simulink model "System_HybridMotorcycle_v1_Wit"  (R2014a)
settings: Solver=ode15s  StartTime=0.0  StopTime=100  RelTol=1e-3
InitFcn:
  | HybridOn=30;
  | SpdHist=3;
undefined symbols (not defined in the file): Acid, HEV_Param, Kt, Kt_Temps, Lead, sigbuilder_block, theta_f, theta_init
libraries: fl_lib x61, nesl_utility x33, sdl_lib x6, LeadAcidBattery_lib x6, simulink x1, electricdrivelib x1, elec_lib x1
(part 2 of 2)

== system System_HybridMotorcycle_v1_Wit/Torque Based Vehicle /Kph Demand/10-15 mode  ==
  Demux : Demux  Tag=STV Demux  Outputs=2
  FromWs : FromWorkspace  Tag=STV FromWs  VariableName=tuvar  SampleTime=0
      SigBuilderData=|
      | common.afterFinalStr = 'Extrapolate'
      | common.sampleTime = '0'
      | dataSet.timeRange = [0 660]
      | dataSet.name = '10-15 Mode Cycle'
      | sbobj.Groups.Name = '10-15 Mode Cycle'
      | sbobj.Groups.Signals(1).Name = 'Target speed'
      | sbobj.Groups.Signals(1).XData = [0 44 51 73 73 89 103 118 128 130 142 152 159 179 186 201 208 224 238 253 263 265 277 287 294 314 321 336 343 359 373 388 398 400 412 422 429 494 512 524 528 532 548 558 569 579 589 593 615 620 640 650 660]
      | sbobj.Groups.Signals(1).YData = [0 0 10 10 0 0 40 40 20 20 40 20 0 0 20 20 0 0 40 40 20 20 40 20 0 0 20 20 0 0 40 40 20 20 40 20 0 0 50 50 40 40 60 60 70 70 50 50 70 70 30 0 0]
      | sbobj.Groups.Signals(2).Name = 'Signal 1'
      | sbobj.Groups.Signals(2).XData = [0 20 120 120 220 220 320 320 420 420 520 520 620 650 660]
      | sbobj.Groups.Signals(2).YData = [0 10 10 20 20 30 30 40 39.8 50 50 60 60 0.5 0]
  Target speed : Outport  Tag=STV Outport
  Signal 1 : Outport  Tag=STV Outport  Port=2
  wires:
  FromWs/1 -> Demux/1
  Demux/1 -> Target speed/1
  Demux/2 -> Signal 1/1

== system System_HybridMotorcycle_v1_Wit/Torque Based Vehicle /MotorGearRatio/AngVel ==
  Ideal Rotational Motion Sensor : fl_lib/Mechanical/Mechanical Sensors/Ideal Rotational Motion Sensor  offset=0 rad
  Mechanical Rotational Reference : fl_lib/Mechanical/Rotational Elements/Mechanical Rotational Reference
  PS-S : nesl_utility/PS-Simulink Converter  PhysicalDomain=network_engine_domain  SubClassName=ps_output  LeftPortType=input  RightPortType=output  PseudoPeriodic=off  Frequencies=[]  Unit=rpm  AffineConversion=off
  Terminator : Terminator
  ang_vel : Scope
      settings: TimeRange=1  YMin=0  YMax=1  SaveName=ScopeData4
  R : PMIOPort  Port=1  Side=Left
  wires:
  [AngVel] -> Terminator/1
  PS-S/1 -> [AngVel], ang_vel/1  "ang_vel"
  connections:
  R/RConn1 -- Ideal Rotational Motion Sensor/LConn1
  Mechanical Rotational Reference/LConn1 -- Ideal Rotational Motion Sensor/RConn1
  Ideal Rotational Motion Sensor/RConn2 -- PS-S/LConn1

== system System_HybridMotorcycle_v1_Wit/Torque Based Vehicle /MotorGearRatio/AngVel1 ==
  Ideal Rotational Motion Sensor : fl_lib/Mechanical/Mechanical Sensors/Ideal Rotational Motion Sensor  offset=0 rad
  Mechanical Rotational Reference : fl_lib/Mechanical/Rotational Elements/Mechanical Rotational Reference
  PS-S : nesl_utility/PS-Simulink Converter  PhysicalDomain=network_engine_domain  SubClassName=ps_output  LeftPortType=input  RightPortType=output  PseudoPeriodic=off  Frequencies=[]  Unit=rpm  AffineConversion=off
  Terminator : Terminator
  ang_vel : Scope
      settings: TimeRange=1  YMin=0  YMax=1  SaveName=ScopeData4
  R : PMIOPort  Port=1  Side=Left
  wires:
  PS-S/1 -> ang_vel/1, [AngVel1]  "ang_vel"
  [AngVel1] -> Terminator/1
  connections:
  Ideal Rotational Motion Sensor/RConn2 -- PS-S/LConn1
  Mechanical Rotational Reference/LConn1 -- Ideal Rotational Motion Sensor/RConn1
  R/RConn1 -- Ideal Rotational Motion Sensor/LConn1

== system System_HybridMotorcycle_v1_Wit/Torque Based Vehicle /MotorGearRatio/Post-Gear Torque Speed Sensor ==
  Ideal Rotational Motion Sensor : fl_lib/Mechanical/Mechanical Sensors/Ideal Rotational Motion Sensor  offset=0 rad
  Ideal Torque Sensor : fl_lib/Mechanical/Mechanical Sensors/Ideal Torque Sensor
  Mechanical Rotational Reference1 : fl_lib/Mechanical/Rotational Elements/Mechanical Rotational Reference
  PS-Simulink Converter1 : nesl_utility/PS-Simulink Converter  PhysicalDomain=network_engine_domain  SubClassName=ps_output  LeftPortType=input  RightPortType=output  PseudoPeriodic=off  Frequencies=[]  Unit=N*m  AffineConversion=off
  PS-Simulink Converter3 : nesl_utility/PS-Simulink Converter  PhysicalDomain=network_engine_domain  SubClassName=ps_output  LeftPortType=input  RightPortType=output  PseudoPeriodic=off  Frequencies=[]  Unit=rpm  AffineConversion=off
  In : PMIOPort  Port=1  Side=Left
  Out : PMIOPort  Port=2  Side=Right
  tag scope: PostGear_Speed=global, PostGear_Torque=global
  wires:
  PS-Simulink Converter3/1 -> [PostGear_Speed]
  PS-Simulink Converter1/1 -> [PostGear_Torque]
  connections:
  Ideal Torque Sensor/RConn1 -- Out/RConn1
  Ideal Rotational Motion Sensor/RConn2 -- PS-Simulink Converter3/LConn1
  PS-Simulink Converter1/LConn1 -- Ideal Torque Sensor/RConn2
  Ideal Rotational Motion Sensor/RConn1 -- Mechanical Rotational Reference1/LConn1
  Ideal Torque Sensor/LConn1 -- In/RConn1 -- Ideal Rotational Motion Sensor/LConn1

== system System_HybridMotorcycle_v1_Wit/Torque Based Vehicle /MotorGearRatio/Pre-Gear Torque Speed Sensor ==
  Ideal Rotational Motion Sensor : fl_lib/Mechanical/Mechanical Sensors/Ideal Rotational Motion Sensor  offset=0 rad
  Ideal Torque Sensor : fl_lib/Mechanical/Mechanical Sensors/Ideal Torque Sensor
  Mechanical Rotational Reference1 : fl_lib/Mechanical/Rotational Elements/Mechanical Rotational Reference
  PS-Simulink Converter1 : nesl_utility/PS-Simulink Converter  PhysicalDomain=network_engine_domain  SubClassName=ps_output  LeftPortType=input  RightPortType=output  PseudoPeriodic=off  Frequencies=[]  Unit=N*m  AffineConversion=off
  PS-Simulink Converter3 : nesl_utility/PS-Simulink Converter  PhysicalDomain=network_engine_domain  SubClassName=ps_output  LeftPortType=input  RightPortType=output  PseudoPeriodic=off  Frequencies=[]  Unit=rpm  AffineConversion=off
  In : PMIOPort  Port=1  Side=Left
  Out : PMIOPort  Port=2  Side=Right
  tag scope: PreGear_Speed=global, PreGear_Torque=global
  wires:
  PS-Simulink Converter3/1 -> [PreGear_Speed]
  PS-Simulink Converter1/1 -> [PreGear_Torque]
  connections:
  Ideal Torque Sensor/RConn1 -- Out/RConn1
  Ideal Rotational Motion Sensor/RConn2 -- PS-Simulink Converter3/LConn1
  PS-Simulink Converter1/LConn1 -- Ideal Torque Sensor/RConn2
  Ideal Rotational Motion Sensor/RConn1 -- Mechanical Rotational Reference1/LConn1
  Ideal Torque Sensor/LConn1 -- Ideal Rotational Motion Sensor/LConn1 -- In/RConn1

== system System_HybridMotorcycle_v1_Wit/Torque Based Vehicle /MotorGearRatio/Torque ==
  Ideal Torque Sensor : fl_lib/Mechanical/Mechanical Sensors/Ideal Torque Sensor
  PS-S : nesl_utility/PS-Simulink Converter  PhysicalDomain=network_engine_domain  SubClassName=ps_output  LeftPortType=input  RightPortType=output  PseudoPeriodic=off  Frequencies=[]  Unit=N*m  AffineConversion=off
  Terminator : Terminator
  torque : Scope
      settings: TimeRange=10  YMin=0  YMax=1
  R : PMIOPort  Port=1  Side=Left
  C : PMIOPort  Port=2  Side=Right
  wires:
  [Torque] -> Terminator/1
  PS-S/1 -> [Torque], torque/1  "torque"
  connections:
  C/RConn1 -- Ideal Torque Sensor/RConn1
  Ideal Torque Sensor/RConn2 -- PS-S/LConn1
  R/RConn1 -- Ideal Torque Sensor/LConn1

== system System_HybridMotorcycle_v1_Wit/Torque Based Vehicle /MotorGearRatio/Torque1 ==
  Ideal Torque Sensor : fl_lib/Mechanical/Mechanical Sensors/Ideal Torque Sensor
  PS-S : nesl_utility/PS-Simulink Converter  PhysicalDomain=network_engine_domain  SubClassName=ps_output  LeftPortType=input  RightPortType=output  PseudoPeriodic=off  Frequencies=[]  Unit=N*m  AffineConversion=off
  Terminator : Terminator
  torque : Scope
      settings: TimeRange=10  YMin=0  YMax=1
  R : PMIOPort  Port=1  Side=Left
  C : PMIOPort  Port=2  Side=Right
  wires:
  PS-S/1 -> torque/1, [Torque1]  "torque"
  [Torque1] -> Terminator/1
  connections:
  R/RConn1 -- Ideal Torque Sensor/LConn1
  Ideal Torque Sensor/RConn2 -- PS-S/LConn1
  C/RConn1 -- Ideal Torque Sensor/RConn1

== system System_HybridMotorcycle_v1_Wit/Torque Based Vehicle /Vehicle Body/AngVel ==
  Ideal Rotational Motion Sensor : fl_lib/Mechanical/Mechanical Sensors/Ideal Rotational Motion Sensor  offset=0 rad
  Mechanical Rotational Reference : fl_lib/Mechanical/Rotational Elements/Mechanical Rotational Reference
  PS-S : nesl_utility/PS-Simulink Converter  PhysicalDomain=network_engine_domain  SubClassName=ps_output  LeftPortType=input  RightPortType=output  PseudoPeriodic=off  Frequencies=[]  Unit=rad/s  AffineConversion=off
  Terminator : Terminator
  ang_vel : Scope
      settings: TimeRange=1  YMin=0  YMax=1  SaveName=ScopeData4
  R : PMIOPort  Port=1  Side=Left
  wires:
  [AngVel] -> Terminator/1
  PS-S/1 -> [AngVel], ang_vel/1  "ang_vel"
  connections:
  R/RConn1 -- Ideal Rotational Motion Sensor/LConn1
  Mechanical Rotational Reference/LConn1 -- Ideal Rotational Motion Sensor/RConn1
  Ideal Rotational Motion Sensor/RConn2 -- PS-S/LConn1

== system System_HybridMotorcycle_v1_Wit/Torque Based Vehicle /Vehicle Body/AngVel1 ==
  Ideal Rotational Motion Sensor : fl_lib/Mechanical/Mechanical Sensors/Ideal Rotational Motion Sensor  offset=0 rad
  Mechanical Rotational Reference : fl_lib/Mechanical/Rotational Elements/Mechanical Rotational Reference
  PS-S : nesl_utility/PS-Simulink Converter  PhysicalDomain=network_engine_domain  SubClassName=ps_output  LeftPortType=input  RightPortType=output  PseudoPeriodic=off  Frequencies=[]  Unit=rad/s  AffineConversion=off
  Terminator : Terminator
  ang_vel : Scope
      settings: TimeRange=1  YMin=0  YMax=1  SaveName=ScopeData4
  R : PMIOPort  Port=1  Side=Left
  wires:
  PS-S/1 -> ang_vel/1, [AngVel1]  "ang_vel"
  [AngVel1] -> Terminator/1
  connections:
  Ideal Rotational Motion Sensor/RConn2 -- PS-S/LConn1
  Mechanical Rotational Reference/LConn1 -- Ideal Rotational Motion Sensor/RConn1
  R/RConn1 -- Ideal Rotational Motion Sensor/LConn1

== stateflow chart System_HybridMotorcycle_v1_Wit/Control Module/Speed State Mode ==
  state Motor_Mode
    entry: Motor_En = 1;
    Engine_En = 0;
  state Engine_Mode
    entry: Motor_En = 0;
    Engine_En = 1;
  (default) -> Motor_Mode
  Engine_Mode -> Motor_Mode : [Vehicle_Speed< ...
      | HybridOn + SpdHist]
  Motor_Mode -> Engine_Mode : [Vehicle_Speed >...
      |  HybridOn - SpdHist]
  data: Vehicle_Speed input; Motor_En output double; Engine_En output double; HybridOn constant double =HybridOn; SpdHist constant double =SpdHist
